simulink model "Boucle_position"  (R2017a)
settings: Solver=VariableStepAuto  StartTime=0.0  StopTime=10.0  RelTol=1e-3
values from neighbouring files (symbols this model uses):
  h = 50e-6    (= 5e-05)    [MotorDat_MSTPM1 (1).m]    (also in ParamMinduction0.m; parametres.m = 1e-05)
  Imax = 9.23    [parametres.m]
  J = 0.004    [MotorDat_MSTPM1 (1).m]    (also in ParamMinduction0.m = 0.006; parametres.m = 0.000131)
  K = 55.4e-3    (= 0.0554)    [parametres.m]
  K2 = 3.9789e-4    (= 0.00039789)    [parametres.m]
  K3 = 10*10^3 / 400    (= 25)    [parametres.m]
  kv = 0    [parametres.m]
  L = 1.7e-3    (= 0.0017)    [MotorDat_MSTPM1 (1).m]    (also in parametres.m = 3.08e-05)
  R = 0.13    [MotorDat_MSTPM1 (1).m]    (also in parametres.m = 0.0809)
  Umax = 24    [parametres.m]
  Xref = 400e-3    (= 0.4)    [parametres.m]
undefined symbols (not defined in the file or in its folder): sigbuilder_block
undefined symbols (not defined in the file): Kii1, Kpi1
libraries: simulink x2
settings Model: Creator=seb  LastModifiedBy=seb

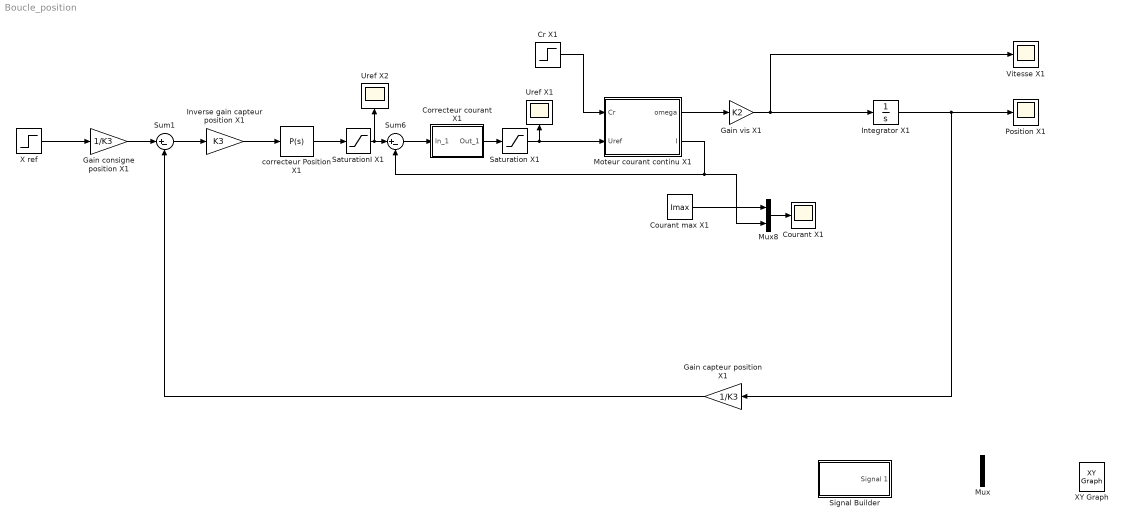
== system Boucle_position ==
  Correcteur courant X1 : Subsystem  AncestorBlock=simulink_extras/Additional Linear/PID Controller  mask(PID Controller){P=Kpi1, I=Kii1, D=0}
      mask prompts: P "Proportional:"; I "Integral:"; D "Derivative:"
      mask help:
      | Enter expressions for proportional, integral, and derivative terms.
      | P+I/s+Ds
      mask Help: This block implements a PID controller where parameters are entered for the Proportional, Integral and Derivative terms. Unmask this block to see how it works. The derivative term is implemented using a true derivative block.
      mask Display: disp('PI')
  Courant X1 : Scope
  Courant max X1 : Constant  Value=Imax
  Cr X1 : Step  Time=0.30  After=0  SampleTime=0
  Gain capteur position X1 : Gain  Gain=1/K3
  Gain consigne position X1 : Gain  Gain=1/K3
  Gain vis X1 : Gain  Gain=K2
  Integrator X1 : Integrator
  Inverse gain capteur position X1 : Gain  Gain=K3
  Moteur courant continu X1 : Subsystem
  Mux : Mux  Inputs=2
  Mux8 : Mux  Inputs=2
  Position X1 : Scope
  Saturation X1 : Saturate  UpperLimit=Umax  LowerLimit=-Umax
  SaturationI X1 : Saturate  UpperLimit=Imax  LowerLimit=-Imax
  Signal Builder : Subsystem  Tag=STV Subsys  LoadFcn=sigbuilder_block('load');  StartFcn=sigbuilder_block('start');  StopFcn=sigbuilder_block('stop');  ClipboardFcn=sigbuilder_block('clipboard');  mask(Sigbuilder block){tuvar=[0:10]}
      mask help: Simulink:masks:SigbuilderBlock_MD
      mask init:
      | if ~strcmp(get_param(bdroot(gcbh),'SimulationStatus'),'stopped') tuvar = sigbuilder_block('maskInit'); end
      settings: CopyFcn=sigbuilder_block('copy');  DeleteFcn=sigbuilder_block('delete');  ModelCloseFcn=sigbuilder_block('modelClose');  PreSaveFcn=sigbuilder_block('preSave');  PauseFcn=sigbuilder_block('pause');  ContinueFcn=sigbuilder_block('continue');  NameChangeFcn=sigbuilder_block('namechange');  OpenFcn=sigbuilder_block('open',[437.6 199.2 550.4 400 ]);  CloseFcn=sigbuilder_block('close');
      mask Display: plot(0, 0, 100, 100,[2, 2, 32, 32, 2], [68, 8, 8, 68, 68],[32, 2], [38, 38], [32, 19, 2],[53, 60, 44], [32, 17, 17, 2],[16, 16, 31, 31]);txt = getActiveGroup(gcbh);text(2, 100, txt,'verticalAlignment', 'top');
  Sum1 : Sum  Inputs=|+-
  Sum6 : Sum  Inputs=|+-
  Uref X1 : Scope
  Uref X2 : Scope
  Vitesse X1 : Scope
  X ref : Step  Time=0.2  After=Xref  SampleTime=0
  XY Graph : simulink/Sinks/XY Graph  xmin=-1  xmax=1  ymin=-1  ymax=1  st=-1
  correcteur Position X1 : simulink/Continuous/PID Controller  Controller=P  TimeDomain=Continuous-time  SampleTime=-1  IntegratorMethod=Forward Euler  FilterMethod=Forward Euler  Form=Parallel  UseFilter=on  ControllerParametersSource=internal  P=15  I=75  D=1619.47145027266  N=31076.4779016831  InitialConditionSource=internal  InitialConditionForIntegrator=0  InitialConditionForFilter=0  ExternalReset=none  LimitOutput=off  UpperSaturationLimit=inf  LowerSaturationLimit=-inf  LinearizeAsGain=on  AntiWindupMode=none  Kb=1  TrackingMode=off  Kt=1  PParamMin=[]  PParamMax=[]  IParamMin=[]  IParamMax=[]  DParamMin=[]  DParamMax=[]  NParamMin=[]  NParamMax=[]  KbParamMin=[]  KbParamMax=[]  KtParamMin=[]  KtParamMax=[]  POutMin=[]  POutMax=[]  IOutMin=[]  IOutMax=[]  DOutMin=[]  DOutMax=[]  NOutMin=[]  NOutMax=[]  KbOutMin=[]  KbOutMax=[]  KtOutMin=[]  KtOutMax=[]  IntegratorOutMin=[]  IntegratorOutMax=[]  FilterOutMin=[]  FilterOutMax=[]  SumOutMin=[]  SumOutMax=[]  SumI1OutMin=[]  SumI1OutMax=[]  SumI2OutMin=[]  SumI2OutMax=[]  SumI3OutMin=[]  SumI3OutMax=[]  SumDOutMin=[]  SumDOutMax=[]  SaturationOutMin=[]  SaturationOutMax=[]  IntegratorContinuousStateAttributes=''  IntegratorStateMustResolveToSignalObject=off  IntegratorRTWStateStorageClass=Auto  FilterContinuousStateAttributes=''  FilterStateMustResolveToSignalObject=off  FilterRTWStateStorageClass=Auto  DifferentiatorICPrevScaledInput=0  DifferentiatorOutMin=[]  DifferentiatorOutMax=[]  InitialConditionSetting=State (most efficient)
  wires:
  Correcteur courant X1/1(Out_1) -> Saturation X1/1
  Moteur courant continu X1/2(I) -> Mux8/2, Sum6/2
  Moteur courant continu X1/1(omega) -> Gain vis X1/1
  correcteur Position X1/1 -> SaturationI X1/1
  Saturation X1/1 -> Moteur courant continu X1/2(Uref), Uref X1/1
  Sum6/1 -> Correcteur courant X1/1(In_1)
  SaturationI X1/1 -> Uref X2/1, Sum6/1
  Courant max X1/1 -> Mux8/1
  Cr X1/1 -> Moteur courant continu X1/1(Cr)
  Gain vis X1/1 -> Vitesse X1/1, Integrator X1/1
  Integrator X1/1 -> Gain capteur position X1/1, Position X1/1
  Mux8/1 -> Courant X1/1
  Gain capteur position X1/1 -> Sum1/2
  X ref/1 -> Gain consigne position X1/1
  Sum1/1 -> Inverse gain capteur position X1/1
  Gain consigne position X1/1 -> Sum1/1
  Inverse gain capteur position X1/1 -> correcteur Position X1/1

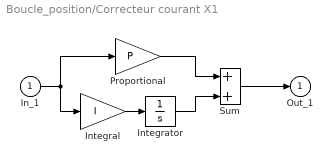
== system Boucle_position/Correcteur courant X1 ==
  In_1 : Inport
  Integral : Gain  Gain=I  SaturateOnIntegerOverflow=on  OutDataTypeStr=Inherit: Same as input  ParamDataTypeStr=Inherit: Same as input
  Integrator : Integrator  LimitOutput=on  UpperSaturationLimit=Umax  LowerSaturationLimit=-Umax
  Proportional : Gain  Gain=P  SaturateOnIntegerOverflow=on  OutDataTypeStr=Inherit: Same as input  ParamDataTypeStr=Inherit: Same as input
  Sum : Sum  SaturateOnIntegerOverflow=on  InputSameDT=on  OutDataTypeStr=Inherit: Same as first input
  Out_1 : Outport  InitialOutput=0
  wires:
  Proportional/1 -> Sum/1
  In_1/1 -> Proportional/1, Integral/1
  Integrator/1 -> Sum/2
  Integral/1 -> Integrator/1
  Sum/1 -> Out_1/1

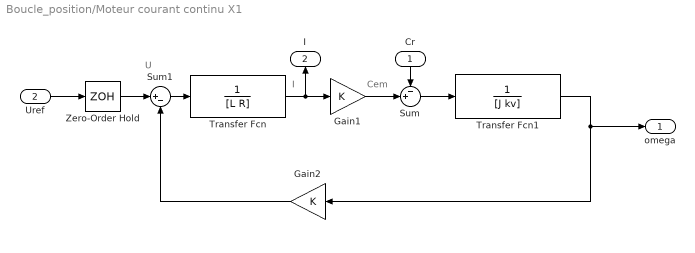
== system Boucle_position/Moteur courant continu X1 ==
  note: U
  note: I
  note: Cem
  Cr : Inport
  Uref : Inport  Port=2
  Gain1 : Gain  Gain=K
  Gain2 : Gain  Gain=K
  Sum : Sum  Inputs=-+|
  Sum1 : Sum  Inputs=|+-
  Transfer Fcn : TransferFcn  Denominator=[L R]
  Transfer Fcn1 : TransferFcn  Denominator=[J kv]
  Zero-Order Hold : ZeroOrderHold  SampleTime=h
  omega : Outport
  I : Outport  Port=2
  wires:
  Transfer Fcn/1 -> I/1, Gain1/1
  Gain1/1 -> Sum/2
  Sum/1 -> Transfer Fcn1/1
  Transfer Fcn1/1 -> Gain2/1, omega/1
  Sum1/1 -> Transfer Fcn/1
  Gain2/1 -> Sum1/2
  Cr/1 -> Sum/1
  Uref/1 -> Zero-Order Hold/1
  Zero-Order Hold/1 -> Sum1/1

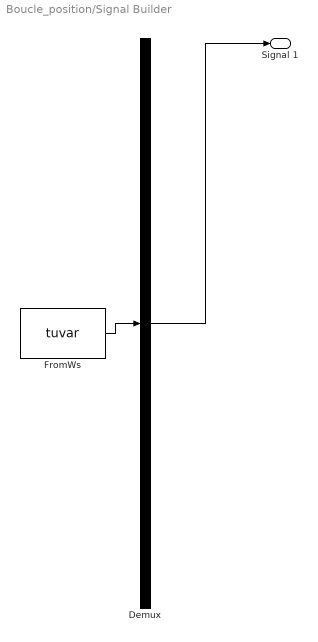
== system Boucle_position/Signal Builder ==
  Demux : Demux  Tag=STV Demux  Outputs=1
  FromWs : FromWorkspace  Tag=STV FromWs  VariableName=tuvar  SampleTime=0
      SigBuilderData=|
      | common.afterFinalStr = 'Extrapolate'
      | common.sampleTime = 0
      | dataSet.timeRange = [0 10]
      | dataSet.name = 'Group 1'
      | sbobj.Groups.Name = 'Group 1'
      | sbobj.Groups.Signals.Name = 'Signal 1'
      | sbobj.Groups.Signals.XData = [0 4 6 6 10]
      | sbobj.Groups.Signals.YData = [0 1 1 0.64 0]
  Signal 1 : Outport  Tag=STV Outport
  wires:
  Demux/1 -> Signal 1/1
  FromWs/1 -> Demux/1
